simulink model "phase1_LC_Control_CIM_Noadapt"  (R2024a)
settings: Solver=FixedStepAuto  StartTime=0.0  StopTime=6  FixedStep=1e-5  MaxStep=1e-6  RelTol=1e-6
values from neighbouring files (symbols this model uses):
  Cf = 22e-6    (= 2.2e-05)    [phase1_LC_Control_CIM_adapt_init.m]    (also in phase1_LC_Control_CIM_noadapt_init.m)
  dcg = dcgain(v2u)    [phase1_LC_Control_CIM_adapt_init.m]    (also in phase1_LC_Control_CIM_noadapt_init.m)
  freq0var = freq0*3    (= 3)    [phase1_LC_Control_CIM_adapt_init.m]    (also in phase1_LC_Control_CIM_noadapt_init.m)
  L1 = 150e-6    (= 0.00015)    [phase1_LC_Control_CIM_adapt_init.m]    (also in phase1_LC_Control_CIM_noadapt_init.m)
  R1 = 0.045    [phase1_LC_Control_CIM_adapt_init.m]    (also in phase1_LC_Control_CIM_noadapt_init.m)
  Rd = 1    [phase1_LC_Control_CIM_adapt_init.m]    (also in phase1_LC_Control_CIM_noadapt_init.m)
  w = 2*pi*freq    (= 6.28318530718)    [phase1_LC_Control_CIM_adapt_init.m]    (also in phase1_LC_Control_CIM_noadapt_init.m)
libraries: spsSeriesRLCBranchLib x3, spsVoltageMeasurementLib x3, spsControlledVoltageSourceLib x2, spsCurrentMeasurementLib x1, cstblocks x1, sps_lib x1
settings Model: Creator=aleks  LastModifiedBy=aleks
settings DataIOCC: ReturnWorkspaceOutputs=off
settings SimscapeCC: SimscapeLogType=all  SimscapeLogOpenViewer=on  SimscapeLogLimitData=off

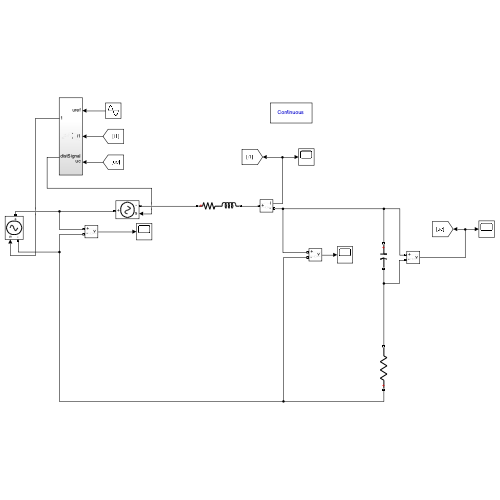
[thumbnail: Simulink's stored preview of the top-level diagram]
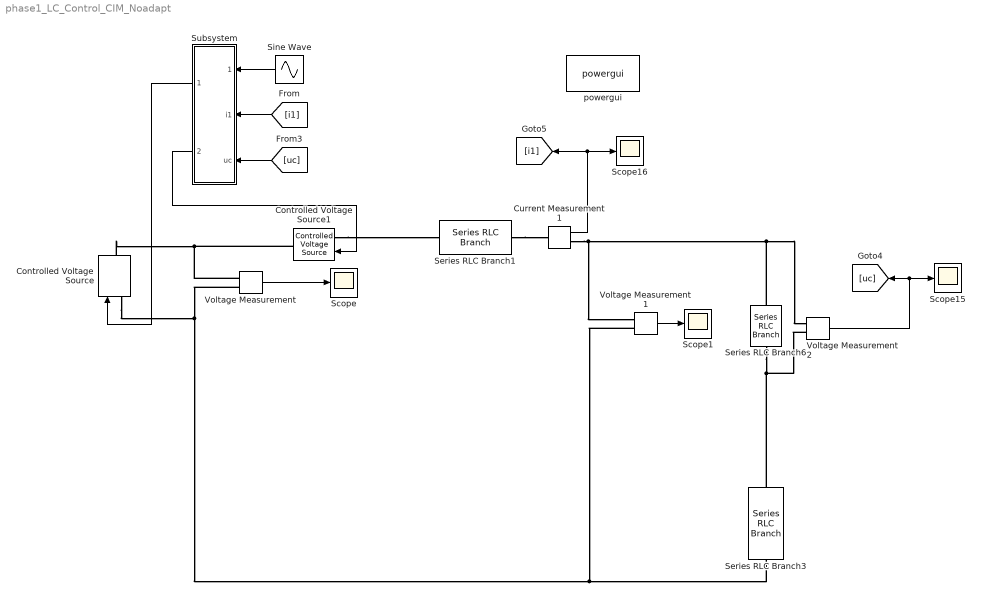
== system phase1_LC_Control_CIM_Noadapt ==
  Controlled Voltage Source : spsControlledVoltageSourceLib/Controlled Voltage Source  Initialize=on  Source_Type=AC  Amplitude=0  Phase=0  Frequency=0  Measurements=None
  Controlled Voltage Source1 : spsControlledVoltageSourceLib/Controlled Voltage Source  Initialize=on  Source_Type=AC  Amplitude=0  Phase=0  Frequency=0  Measurements=None
  Current Measurement1 : spsCurrentMeasurementLib/Current Measurement  PhasorSimulation=off  OutputType=Complex  PSBequivalent=0
  Scope{,1,15..16} (4 alike) : Scope
  Series RLC Branch1 : spsSeriesRLCBranchLib/Series RLC Branch  LConnTagsString=__new0  RConnTagsString=__new0  BranchType=RL  Resistance=R1  Inductance=L1  SetiL0=off  InitialCurrent=0  Capacitance=1e-6  Setx0=off  InitialVoltage=0  Measurements=None
  Series RLC Branch3 : spsSeriesRLCBranchLib/Series RLC Branch  LConnTagsString=__new0  RConnTagsString=__new0  BranchType=R  Resistance=Rd  Inductance=500e-6  SetiL0=off  InitialCurrent=0  Capacitance=Cf  Setx0=off  InitialVoltage=0  Measurements=None
  Series RLC Branch6 : spsSeriesRLCBranchLib/Series RLC Branch  LConnTagsString=__new0  RConnTagsString=__new0  BranchType=C  Resistance=Rd  Inductance=500e-6  SetiL0=off  InitialCurrent=0  Capacitance=Cf  Setx0=off  InitialVoltage=0  Measurements=None
  Sine Wave : Sin  Amplitude=15/dcg  Frequency=w  SampleTime=0
  Subsystem : Subsystem
  Voltage Measurement : spsVoltageMeasurementLib/Voltage Measurement  PhasorSimulation=off  OutputType=Complex  PSBequivalent=0
  Voltage Measurement1 : spsVoltageMeasurementLib/Voltage Measurement  PhasorSimulation=off  OutputType=Complex  PSBequivalent=0
  Voltage Measurement2 : spsVoltageMeasurementLib/Voltage Measurement  PhasorSimulation=off  OutputType=Complex  PSBequivalent=0
  powergui : sps_lib/powergui  Priority=1  SimulationMode=Continuous  SampleTime=10e-6  frequency=60  Iterations=50  frequencyindice=0  Pbase=100e6  ErrMax=1e-4  UnitsV=kV  UnitsW=MW  buscounter=0  FunctionMessages=off  echomessages=off  EnableUseOfTLC=off  CurrentSourceSwitches=off  DisableSnubberDevices=off  DisableRonSwitches=off  DisableVfSwitches=off  DisplayEquations=off  AutomaticDiscreteSolvers=off  SolverType=Tustin/Backward Euler (TBE)  Interpol=off  ExternalGateDelay=off  methode=off  Ts=100  x0status=blocks  SPID=on  SwTol=0  HookPort=off  NonlinearTolerance=1e-4  nMaxIteration=100  ContinueOnMaxIteration=off  RestoreLinks=warning  ResistiveCurrentMeasurement=off  Frange=[0:2:500]  Ylog=off  Xlog=on  ShowGrid=off  save=off  variable=ZData  structure=0  ZoomFFT=off  StartTime=0.0  cycles=1  DisplayStyle=1  fundamental=60  FreqAxis=off  MaxFrequency=1000  frequencyindicesteady=1  RmsSteady=1  display=off
  wires:
  Voltage Measurement/1 -> Scope/1
  Subsystem/1(1) -> Controlled Voltage Source/1
  [i1] -> Subsystem/2(i1)
  [uc] -> Subsystem/3(uc)
  Voltage Measurement2/1 -> Scope15/1, [uc]
  Current Measurement1/1 -> Scope16/1, [i1]
  Voltage Measurement1/1 -> Scope1/1
  Sine Wave/1 -> Subsystem/1(uref)
  Subsystem/2(distSignal) -> Controlled Voltage Source1/1
  connections:
  Voltage Measurement/LConn1 -- Controlled Voltage Source1/RConn1 -- Controlled Voltage Source/RConn1
  Voltage Measurement/LConn2 -- Controlled Voltage Source/LConn1 -- Series RLC Branch3/LConn1 -- Voltage Measurement1/LConn2
  Series RLC Branch1/RConn1 -- Current Measurement1/LConn1
  Voltage Measurement2/LConn2 -- Series RLC Branch3/RConn1 -- Series RLC Branch6/RConn1
  Current Measurement1/RConn1 -- Voltage Measurement1/LConn1 -- Series RLC Branch6/LConn1 -- Voltage Measurement2/LConn1
  Controlled Voltage Source1/LConn1 -- Series RLC Branch1/LConn1

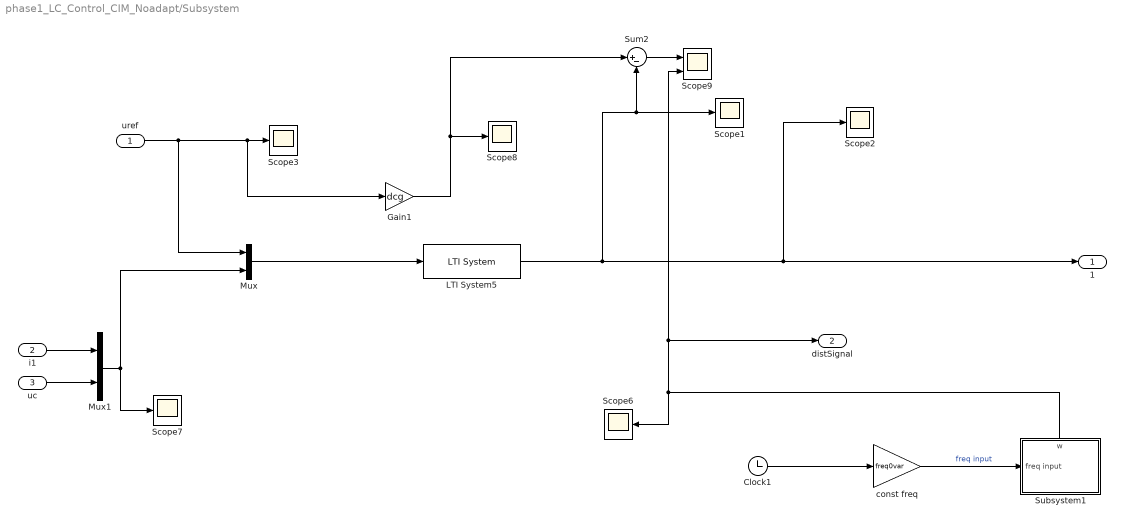
== system phase1_LC_Control_CIM_Noadapt/Subsystem ==
  uref : Inport
  i1 : Inport  Port=2
  uc : Inport  Port=3
  Clock1 : Clock
  Gain1 : Gain  Gain=dcg
  LTI System5 : cstblocks/LTI System  sys=SFControl  IC=[]  PadeOrder=0
  Mux : Mux  Inputs=2
  Mux1 : Mux  Inputs=2
  Scope{1..3,6..8} (6 alike) : Scope
  Scope9 : Scope  NumInputPorts=2
  Subsystem1 : Subsystem
      settings: PortSchema="{\"entries\":[{\"content\":{\"sides\":[{\"content\":{\"connectorIds\":[\"In1\"]},\"type\":\"ConnectorPlacement.EquallySpacedRectSide\",\"uuid\":\"8bb38228-3bfd-4ae6-808e-88de23dff197\"},{\"content\":{\"side\":\"RIGHT\"},\"type\":\"ConnectorPlacement.EquallySpacedRectSide\",\"uuid\":\"838e29f9-37df-4c86-a8f7-90e289e1c513\"},{\"content\":{\"connectorIds\":[\"Out1\"],\"side\":\"TOP\"},\"type\":\"ConnectorPlacement.EquallySpacedRectSide\",\"uuid\":\"6e4fecd3-8130-46cd-a081-09e68c069565\"}]},\"type\":\"ConnectorPlacement.EquallySpacedConnector\",\"uuid\":\"764d7bec-48d4-42ac-bbe4-5dd81e7c6ed5\"}],\"packageUris\":[\"http://schema.mathworks.com/mf0/Connector/R2020b\"],\"version\":\"1.0\"}"
  Sum2 : Sum  Inputs=|+-
  const freq : Gain  Gain=freq0var
  1 : Outport
  distSignal : Outport  Port=2
  wires:
  LTI System5/1 -> 1/1, Scope2/1, Sum2/2, Scope1/1
  uc/1 -> Mux1/2
  i1/1 -> Mux1/1
  Mux/1 -> LTI System5/1
  uref/1 -> Mux/1, Gain1/1, Scope3/1
  Mux1/1 -> Mux/2, Scope7/1
  Clock1/1 -> const freq/1
  Subsystem1/1(w) -> Scope6/1, distSignal/1, Scope9/2
  Gain1/1 -> Sum2/1, Scope8/1
  Sum2/1 -> Scope9/1
  const freq/1 -> Subsystem1/1(freq input)  "freq input"

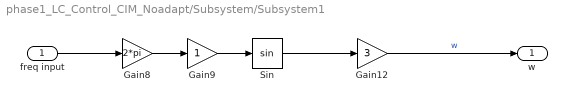
== system phase1_LC_Control_CIM_Noadapt/Subsystem/Subsystem1 ==
  freq input : Inport
  Gain12 : Gain  Gain=3
  Gain8 : Gain  Gain=2*pi
  Gain9 : Gain
  Sin : Trigonometry
  w : Outport
  wires:
  Gain12/1 -> w/1  "w"
  Gain9/1 -> Sin/1
  freq input/1 -> Gain8/1
  Sin/1 -> Gain12/1
  Gain8/1 -> Gain9/1
